simulink model "MSDR_and_BOP_v1_1"  (R2019a)
settings: Solver=ode45  StartTime=0.0  StopTime=15000  FixedStep=0.1  MaxStep=10
values from neighbouring files (symbols this model uses):
  a_f = -3.22E-5    (= -3.22e-05)    [MSDR_parameters_v1_1.m]
  a_g = +2.35E-5    (= 2.35e-05)    [MSDR_parameters_v1_1.m]
  A_s = 1.2245    [MSDR_parameters_v1_1.m]
  beta = [0.000223, 0.001457, 0.001307, 0.002628, 0.000766, 0.000280]    [MSDR_parameters_v1_1.m]
  beta_t = sum(beta)    [MSDR_parameters_v1_1.m]
  ce1 = 1.2471e-07    [MSDR_parameters_v1_1.m]
  ce2 = 5.3816e-14    [MSDR_parameters_v1_1.m]
  ce3 = 3.3721e-08    [MSDR_parameters_v1_1.m]
  Cp_fw = 3200.448e-6    (= 0.003200448)    [MSDR_parameters_v1_1.m]
  Cp_hr = 0.0021520    (= 0.002152)    [MSDR_parameters_v1_1.m]
  Cp_p = Cp_s_shx    (= 0.00154912)    [MSDR_parameters_v1_1.m]
  Cp_s = Cp_s*1e-6    (= 3.588208e-09)    [MSDR_parameters_v1_1.m]
  Cp_s_shx = 1549.12e-6    (= 0.00154912)    [MSDR_parameters_v1_1.m]
  Cp_sc = 4761.392e-6    (= 0.004761392)    [MSDR_parameters_v1_1.m]
  Cp_w = 456.056e-6    (= 0.000456056)    [MSDR_parameters_v1_1.m]
  D_it = 0.0141478    [MSDR_parameters_v1_1.m]
  D_ot = 0.015875    [MSDR_parameters_v1_1.m]
  dHs_dPs = -0.042433622114357    (= -0.0424336221144)    [MSDR_parameters_v1_1.m]
  eta_hp_isen = 0.861    [MSDR_parameters_v1_1.m]
  eta_lp_isen = 0.861    [MSDR_parameters_v1_1.m]
  gamma_I = 5.1135e-2    (= 0.051135)    [MSDR_parameters_v1_1.m]
  gamma_Xe = 1.1628e-2    (= 0.011628)    [MSDR_parameters_v1_1.m]
  H_fwh1 = 0.46009    [MSDR_parameters_v1_1.m]
  h_fwh1 = 0.5927    [MSDR_parameters_v1_1.m]
  H_fwh2 = 0.6784    [MSDR_parameters_v1_1.m]
  h_fwh2 = 0.5927    [MSDR_parameters_v1_1.m]
  H_lp_isen = 958.4*1054.35e-6/0.45359237    (= 2.22774699671)    [MSDR_parameters_v1_1.m]
  H_nc = 3.2952    [MSDR_parameters_v1_1.m]
  h_pw = h_s_shx    (= 0.00567446)    [MSDR_parameters_v1_1.m]
  H_rh = 2.8115    [MSDR_parameters_v1_1.m]
  h_wb = 13349.334646671E-6    (= 0.0133493346467)    [MSDR_parameters_v1_1.m]
  h_ws = 5732.378387768E-6    (= 0.00573237838777)    [MSDR_parameters_v1_1.m]
  h_wsc = 8385.005556375E-6    (= 0.00838500555638)    [MSDR_parameters_v1_1.m]
  hA_fg = [h_fg*A_fg/2, h_fg*A_fg/2]    [MSDR_parameters_v1_1.m]
  hA_p_phx1 = h_p_phx*A_p_phx    [MSDR_parameters_v1_1.m]
  hA_p_phx2 = h_p_phx*A_p_phx    [MSDR_parameters_v1_1.m]
  hA_p_phx3 = h_p_phx*A_p_phx    [MSDR_parameters_v1_1.m]
  hA_p_phx4 = h_p_phx*A_p_phx    [MSDR_parameters_v1_1.m]
  hA_p_phx5 = h_p_phx*A_p_phx    [MSDR_parameters_v1_1.m]
  hA_p_phx6 = h_p_phx*A_p_phx    [MSDR_parameters_v1_1.m]
  hA_p_shx1 = h_p_shx*A_p_shx    [MSDR_parameters_v1_1.m]
  hA_p_shx2 = h_p_shx*A_p_shx    [MSDR_parameters_v1_1.m]
  hA_p_shx3 = h_p_shx*A_p_shx    [MSDR_parameters_v1_1.m]
  hA_p_shx4 = h_p_shx*A_p_shx    [MSDR_parameters_v1_1.m]
  hA_p_shx5 = h_p_shx*A_p_shx    [MSDR_parameters_v1_1.m]
  hA_p_shx6 = h_p_shx*A_p_shx    [MSDR_parameters_v1_1.m]
  hA_s_phx1 = h_s_phx*A_s_phx    [MSDR_parameters_v1_1.m]
  hA_s_phx2 = h_s_phx*A_s_phx    [MSDR_parameters_v1_1.m]
  hA_s_phx3 = h_s_phx*A_s_phx    [MSDR_parameters_v1_1.m]
  hA_s_phx4 = h_s_phx*A_s_phx    [MSDR_parameters_v1_1.m]
  hA_s_phx5 = h_s_phx*A_s_phx    [MSDR_parameters_v1_1.m]
  hA_s_phx6 = h_s_phx*A_s_phx    [MSDR_parameters_v1_1.m]
  hA_s_shx1 = h_s_shx*A_s_shx    [MSDR_parameters_v1_1.m]
  hA_s_shx2 = h_s_shx*A_s_shx    [MSDR_parameters_v1_1.m]
  hA_s_shx3 = h_s_shx*A_s_shx    [MSDR_parameters_v1_1.m]
  hA_s_shx4 = h_s_shx*A_s_shx    [MSDR_parameters_v1_1.m]
  hA_s_shx5 = h_s_shx*A_s_shx    [MSDR_parameters_v1_1.m]
  hA_s_shx6 = h_s_shx*A_s_shx    [MSDR_parameters_v1_1.m]
  I_0 = gamma_I*Sig_f_msdr*phi_0/lam_I    (= 4.38204721773e+16)    [MSDR_parameters_v1_1.m]
  Ifa = [0.25, 0.25]    [MSDR_parameters_v1_1.m]
  Ifb = [0.25, 0.25]    [MSDR_parameters_v1_1.m]
  Ig = [0.5, 0.5]    [MSDR_parameters_v1_1.m]
  K_1 = 11.632248097704855    (= 11.6322480977)    [MSDR_parameters_v1_1.m]
  K_4 = b(1)    [MSDR_parameters_v1_1.m]
  K_5 = a(1)    [MSDR_parameters_v1_1.m]
  K_b = 12.834854076292217    (= 12.8348540763)    [MSDR_parameters_v1_1.m]
  K_b_hp = 0.1634    [MSDR_parameters_v1_1.m]
  K_b_lp = 0.2174    [MSDR_parameters_v1_1.m]
  K_sc = -17.615718797133468    (= -17.6157187971)    [MSDR_parameters_v1_1.m]
  ka = [0.235, 0.235]    [MSDR_parameters_v1_1.m]
  kb = [0.235, 0.235]    [MSDR_parameters_v1_1.m]
  kga = [0.015, 0.015]    [MSDR_parameters_v1_1.m]
  kgb = [0.015, 0.015]    [MSDR_parameters_v1_1.m]
  L = 8.5344    [MSDR_parameters_v1_1.m]
  L_b = 2.3645    [MSDR_parameters_v1_1.m]
  L_s = 4.723    [MSDR_parameters_v1_1.m]
  Lam = 2.400E-04    (= 0.00024)    [MSDR_parameters_v1_1.m]
  lam = [0.0124, 0.0305, 0.111, 0.301, 1.14, 3.01]    [MSDR_parameters_v1_1.m]
  lam_bubl = 2.0e-2    (= 0.02)    [MSDR_parameters_v1_1.m]
  lam_I = 2.875e-5    (= 2.875e-05)    [MSDR_parameters_v1_1.m]
  lam_Xe = 2.0916e-5    (= 2.0916e-05)    [MSDR_parameters_v1_1.m]
  m_3m = W_3*2    (= 8618.207327)    [MSDR_parameters_v1_1.m]
  m_fm = W_f*2    (= 9978.96)    [MSDR_parameters_v1_1.m]
  m_sb = 1717    [MSDR_parameters_v1_1.m]
  M_stm = 0.018    [MSDR_parameters_v1_1.m]
  mb_cpb = 2.689619410657651e+00    (= 2.68961941066)    [MSDR_parameters_v1_1.m]
  mcp_fa = mfa*Cp_f    [MSDR_parameters_v1_1.m]
  mcp_fb = mfb*Cp_f    [MSDR_parameters_v1_1.m]
  mcp_g = mg*Cp_g    [MSDR_parameters_v1_1.m]
  mcp_p_phx1 = Cp_p_phx*mp_phx1    [MSDR_parameters_v1_1.m]
  mcp_p_phx2 = Cp_p_phx*mp_phx2    [MSDR_parameters_v1_1.m]
  mcp_p_phx3 = Cp_p_phx*mp_phx3    [MSDR_parameters_v1_1.m]
  mcp_p_phx4 = Cp_p_phx*mp_phx4    [MSDR_parameters_v1_1.m]
  mcp_p_phx5 = Cp_p_phx*mp_phx5    [MSDR_parameters_v1_1.m]
  mcp_p_phx6 = Cp_p_phx*mp_phx6    [MSDR_parameters_v1_1.m]
  mcp_p_shx1 = Cp_p_shx*mp_shx1    [MSDR_parameters_v1_1.m]
  mcp_p_shx2 = Cp_p_shx*mp_shx2    [MSDR_parameters_v1_1.m]
  mcp_p_shx3 = Cp_p_shx*mp_shx3    [MSDR_parameters_v1_1.m]
  mcp_p_shx4 = Cp_p_shx*mp_shx4    [MSDR_parameters_v1_1.m]
  mcp_p_shx5 = Cp_p_shx*mp_shx5    [MSDR_parameters_v1_1.m]
  mcp_p_shx6 = Cp_p_shx*mp_shx6    [MSDR_parameters_v1_1.m]
  mcp_s_phx1 = Cp_s_phx*ms_phx1    [MSDR_parameters_v1_1.m]
  mcp_s_phx2 = Cp_s_phx*ms_phx2    [MSDR_parameters_v1_1.m]
  mcp_s_phx3 = Cp_s_phx*ms_phx3    [MSDR_parameters_v1_1.m]
  mcp_s_phx4 = Cp_s_phx*ms_phx4    [MSDR_parameters_v1_1.m]
  mcp_s_phx5 = Cp_s_phx*ms_phx5    [MSDR_parameters_v1_1.m]
  mcp_s_phx6 = Cp_s_phx*ms_phx6    [MSDR_parameters_v1_1.m]
  mcp_s_shx1 = Cp_s_shx*ms_shx1    [MSDR_parameters_v1_1.m]
  mcp_s_shx2 = Cp_s_shx*ms_shx1    [MSDR_parameters_v1_1.m]
  mcp_s_shx3 = Cp_s_shx*ms_shx1    [MSDR_parameters_v1_1.m]
  mcp_s_shx4 = Cp_s_shx*ms_shx1    [MSDR_parameters_v1_1.m]
  mcp_s_shx5 = Cp_s_shx*ms_shx1    [MSDR_parameters_v1_1.m]
  mcp_s_shx6 = Cp_s_shx*ms_shx1    [MSDR_parameters_v1_1.m]
  mcp_t_phx1 = Cp_t_phx*mt_phx1    [MSDR_parameters_v1_1.m]
  mcp_t_phx2 = Cp_t_phx*mt_phx2    [MSDR_parameters_v1_1.m]
  mcp_t_phx3 = Cp_t_phx*mt_phx3    [MSDR_parameters_v1_1.m]
  mcp_t_phx4 = Cp_t_phx*mt_phx4    [MSDR_parameters_v1_1.m]
  mcp_t_phx5 = Cp_t_phx*mt_phx5    [MSDR_parameters_v1_1.m]
  mcp_t_phx6 = Cp_t_phx*mt_phx6    [MSDR_parameters_v1_1.m]
  mcp_t_shx1 = Cp_t_phx*mt_shx1    [MSDR_parameters_v1_1.m]
  ... (+177 more)
undefined symbols (not defined in the file or in its folder): C0, H_con_table, H_convap_table, H_rh_table, H_rh_table1, H_rh_table2, H_rhvap_table, H_s_table, H_table, hA_p_thx1, hA_p_thx2, hA_p_thx3, hA_s_thx1, hA_s_thx2, hA_s_thx3, ln, mcp_p_thx1, mcp_p_thx2, mcp_p_thx3, mcp_s_thx1, mcp_s_thx2, mcp_s_thx3, mcp_t_thx1, mcp_t_thx2, mcp_t_thx3, mp_thx1, mp_thx2, mp_thx3, ms_thx1, ms_thx2, ms_thx3, P_con_table, P_nc_table, P_rh_table, P_rh_table1, pres_table, rho_rh_table, rho_table, SV_nc_table, T0_p_thx1, T0_p_thx2, T0_p_thx3, T0_s_thx1, T0_s_thx2, T0_s_thx3, T0_t_thx1, T0_t_thx2, T0_t_thx3, temp_table, u14, Wp_thx1, Wp_thx2, Wp_thx3, Ws_thx1, Ws_thx2, Ws_thx3
libraries: simulink x10
(part 4 of 4)

== system MSDR_and_BOP_v1_1/HEAT EXCHANGERS/HEAT EXCHANGER LOOP 6/THX2 HEAT TRANSFER ==
  PRIMARY FLUID INLET TEMPERATURE : Inport
  SECONDARY FLUID INLET TEMPERATURE : Inport  Port=2
  PRIMARY FLOW FRACTION : Inport  Port=3
  PRIMARY HEAT TRANSFER FRACTION : Inport  Port=4
  SECONDARY FLOW FRACTION : Inport  Port=5
  SECONDARY HEAT TRANSFER FRACTION : Inport  Port=6
  Mux : Mux  Inputs=16
      settings: DisplayOption=signals
  To Workspace : ToWorkspace  VariableName=thx3_ht  SampleTime=-1
  Tp1_thx3 : Integrator  InitialCondition=T0_p_thx3(1)
  Tp2_thx3 : Integrator  InitialCondition=T0_p_thx3(2)
  "Tp3_thx3 " : Integrator  InitialCondition=T0_p_thx3(3)
  Tp4_thx3 : Integrator  InitialCondition=T0_p_thx3(4)
  Ts1_thx3 : Integrator  InitialCondition=T0_s_thx3(1)
  Ts2_thx3 : Integrator  InitialCondition=T0_s_thx3(2)
  Ts3_thx3 : Integrator  InitialCondition=T0_s_thx3(3)
  Ts4_thx3 : Integrator  InitialCondition=T0_s_thx3(4)
  Tt1_thx3 : Integrator  InitialCondition=T0_t_thx3(1)
  Tt2_thx3 : Integrator  InitialCondition=T0_t_thx3(2)
  d(Tp1_thx3)/dt : Fcn  Expr=(u[13]*Wp_thx3/mp_thx3(1))*(u[1] - u[3]) + (u[14]*hA_p_thx3(1)/mcp_p_thx3(1))*(u[7] - u[3])
  d(Tp2_thx3)/dt : Fcn  Expr=(u[13]*Wp_thx3/mp_thx3(2))*(u[3] - u[4]) + (u[14]*hA_p_thx3(2)/mcp_p_thx3(2))*(u[7] - u[3])
  d(Tp3_thx3)/dt : Fcn  Expr=(u[13]*Wp_thx3/mp_thx3(3))*(u[4] - u[5]) + (u[14]*hA_p_thx3(3)/mcp_p_thx3(3))*(u[8] - u[5])
  d(Tp4_thx3)/dt : Fcn  Expr=(u[13]*Wp_thx3/mp_thx3(4))*(u[5] - u[6]) + (u[14]*hA_p_thx3(4)/mcp_p_thx3(4))*(u[8] - u[5])
  d(Ts1_thx3)/dt : Fcn  Expr=(u[15]*Ws_thx3/ms_thx3(1))*(u[2] - u[9]) + (u[16]*hA_s_thx3(1)/mcp_s_thx3(1))*(u[8] - u[9])
  d(Ts2_thx3)/dt : Fcn  Expr=(u[15]*Ws_thx3/ms_thx3(2))*(u[9] - u[10]) + (u[16]*hA_s_thx3(2)/mcp_s_thx3(2))*(u[8] - u[9])
  d(Ts3_thx3)/dt : Fcn  Expr=(u[15]*Ws_thx3/ms_thx3(3))*(u[10] - u[11]) + (u[16]*hA_s_thx3(3)/mcp_s_thx3(3))*(u[7] - u[11])
  d(Ts4_thx3)/dt : Fcn  Expr=(u[15]*Ws_thx3/ms_thx3(4))*(u[11] - u[12]) + (u[16]*hA_s_thx3(4)/mcp_s_thx3(4))*(u[7] - u[11])
  d(Tt1_thx3)/dt : Fcn  Expr=(u[14]*(hA_p_thx3(1) + hA_p_thx3(2))/mcp_t_thx3(1))*(u[3] - u[7]) + (u[16]*(hA_s_thx3(1) + hA_s_thx3(2))/mcp_t_thx3(1))*(u[11] - u[7])
  d(Tt2_thx3)/dt : Fcn  Expr=(u[14]*(hA_p_thx3(3) + hA_p_thx3(4))/mcp_t_thx3(2))*(u[5] - u[8]) + (u[16]*(hA_s_thx3(3) + hA_s_thx3(4))/mcp_t_thx3(2))*(u[9] - u[8])
  THX3 TEMPERATURES : Outport
  wires:
  Ts1_thx3/1 -> Mux/9
  Ts2_thx3/1 -> Mux/10
  d(Ts2_thx3)/dt/1 -> Ts2_thx3/1
  d(Tp4_thx3)/dt/1 -> Tp4_thx3/1
  Tt1_thx3/1 -> Mux/7
  d(Tp2_thx3)/dt/1 -> Tp2_thx3/1
  Tp4_thx3/1 -> Mux/6
  d(Tt2_thx3)/dt/1 -> Tt2_thx3/1
  SECONDARY FLUID INLET TEMPERATURE/1 -> Mux/2
  Tt2_thx3/1 -> Mux/8
  Mux/1 -> To Workspace/1, THX3 TEMPERATURES/1, d(Ts4_thx3)/dt/1, d(Ts3_thx3)/dt/1, d(Ts2_thx3)/dt/1, d(Ts1_thx3)/dt/1, d(Tt2_thx3)/dt/1, d(Tt1_thx3)/dt/1, d(Tp4_thx3)/dt/1, d(Tp3_thx3)/dt/1, d(Tp2_thx3)/dt/1, d(Tp1_thx3)/dt/1
  d(Tp1_thx3)/dt/1 -> Tp1_thx3/1
  d(Ts4_thx3)/dt/1 -> Ts4_thx3/1
  Tp1_thx3/1 -> Mux/3
  d(Ts1_thx3)/dt/1 -> Ts1_thx3/1
  d(Ts3_thx3)/dt/1 -> Ts3_thx3/1
  Ts3_thx3/1 -> Mux/11
  Ts4_thx3/1 -> Mux/12
  "Tp3_thx3 "/1 -> Mux/5
  d(Tp3_thx3)/dt/1 -> "Tp3_thx3 "/1
  Tp2_thx3/1 -> Mux/4
  d(Tt1_thx3)/dt/1 -> Tt1_thx3/1
  PRIMARY FLUID INLET TEMPERATURE/1 -> Mux/1
  SECONDARY HEAT TRANSFER FRACTION/1 -> Mux/16
  PRIMARY FLOW FRACTION/1 -> Mux/13
  PRIMARY HEAT TRANSFER FRACTION/1 -> Mux/14
  SECONDARY FLOW FRACTION/1 -> Mux/15

== system MSDR_and_BOP_v1_1/HEAT EXCHANGERS/HEAT EXCHANGER LOOP 6/THX3 MATERIAL TRANSPORT ==
  THX3 TEMPERATURES : Inport
  wires:
  THX3 TEMPERATURES/1 -> ?

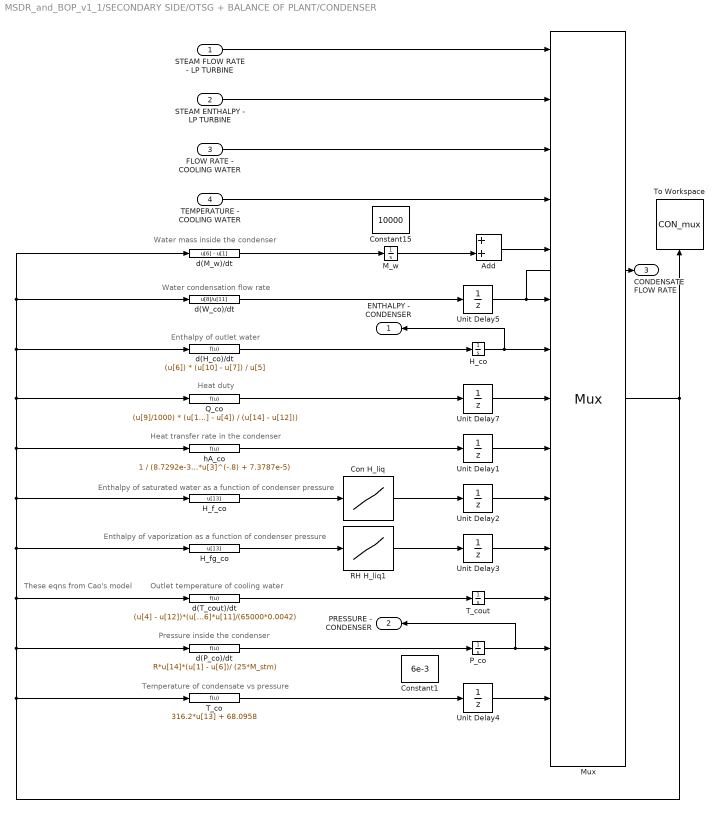
== system MSDR_and_BOP_v1_1/SECONDARY SIDE/OTSG + BALANCE OF PLANT/CONDENSER ==
  note: Water mass inside the condenser
  note: Water condensation flow rate
  note: Enthalpy of outlet water
  note: Heat duty
  note: Heat transfer rate in the condenser
  note: Enthalpy of saturated water as a function of condenser pressure
  note: Enthalpy of vaporization as a function of condenser pressure
  note: Outlet temperature of cooling water
  note: Pressure inside the condenser
  note: Temperature of condensate vs pressure
  note: These eqns from Cao's model
  STEAM FLOW RATE - LP TURBINE : Inport
  STEAM ENTHALPY - LP TURBINE : Inport  Port=2
  FLOW RATE - COOLING WATER : Inport  Port=3
  TEMPERATURE - COOLING WATER : Inport  Port=4
  Add : Sum
  Con H_liq : Lookup_n-D  NumberOfTableDimensions=1  BreakpointsForDimension1=P_con_table  Table=H_con_table  InternalRulePriority=Speed  RndMeth=Simplest  InputSameDT=on
  Constant1 : Constant  Value=6e-3
  Constant15 : Constant  Value=10000
  H_co : Integrator  InitialCondition=.149
  H_f_co : Fcn  Expr=u[13]
  H_fg_co : Fcn  Expr=u[13]
  M_w : Integrator  InitialCondition=10000
  Mux : Mux  Inputs=15
      settings: DisplayOption=signals
  P_co : Integrator  InitialCondition=0.006
  Q_co : Fcn  Expr=(u[9]/1000) * (u[12] - u[4]) / ln((u[14] - u[4]) / (u[14] - u[12]))
  RH H_liq1 : Lookup_n-D  NumberOfTableDimensions=1  BreakpointsForDimension1=P_con_table  Table=H_convap_table  InternalRulePriority=Speed  RndMeth=Simplest  InputSameDT=on
  T_co : Fcn  Expr=316.2*u[13] + 68.0958
  T_cout : Integrator  InitialCondition=40
  To Workspace : ToWorkspace  VariableName=CON_mux  SampleTime=0.1
      settings: Save2DSignal=2-D array (concatenate along first dimension)
  Unit Delay1 : UnitDelay  InitialCondition=140  SampleTime=-1  HasFrameUpgradeWarning=on
  Unit Delay2 : UnitDelay  InitialCondition=0.149  SampleTime=-1  HasFrameUpgradeWarning=on
  Unit Delay3 : UnitDelay  InitialCondition=2.35  SampleTime=-1  HasFrameUpgradeWarning=on
  Unit Delay4 : UnitDelay  InitialCondition=90  SampleTime=-1  HasFrameUpgradeWarning=on
  Unit Delay5 : UnitDelay  InitialCondition=159  SampleTime=-1  HasFrameUpgradeWarning=on
  Unit Delay7 : UnitDelay  InitialCondition=375  SampleTime=-1  HasFrameUpgradeWarning=on
  d(H_co)/dt : Fcn  Expr=(u[6]) * (u[10] - u[7]) / u[5]
  d(M_w)/dt : Fcn  Expr=u[6] - u[1]
  d(P_co)/dt : Fcn  Expr=R*u[14]*(u[1] - u[6])/ (25*M_stm)
  d(T_cout)/dt : Fcn  Expr=(u[4] - u[12])*(u[3]/65000) + u[6]*u[11]/(65000*0.0042)
  d(W_co)/dt : Fcn  Expr=u[8]/u[11]
  hA_co : Fcn  Expr=1 / (8.7292e-3*u[3]^(-.8) + 7.3787e-5)
  ENTHALPY - CONDENSER : Outport
  PRESSURE - CONDENSER : Outport  Port=2
  CONDENSATE FLOW RATE : Outport  Port=3
  wires:
  STEAM FLOW RATE - LP TURBINE/1 -> Mux/1
  d(M_w)/dt/1 -> M_w/1
  STEAM ENTHALPY - LP TURBINE/1 -> Mux/2
  FLOW RATE - COOLING WATER/1 -> Mux/3
  TEMPERATURE - COOLING WATER/1 -> Mux/4
  d(W_co)/dt/1 -> Unit Delay5/1
  Unit Delay5/1 -> CONDENSATE FLOW RATE/1, Mux/6
  d(H_co)/dt/1 -> H_co/1
  H_co/1 -> ENTHALPY - CONDENSER/1, Mux/7
  Unit Delay7/1 -> Mux/8
  Q_co/1 -> Unit Delay7/1
  Unit Delay1/1 -> Mux/9
  hA_co/1 -> Unit Delay1/1
  Unit Delay2/1 -> Mux/10
  H_fg_co/1 -> RH H_liq1/1
  Unit Delay3/1 -> Mux/11
  d(T_cout)/dt/1 -> T_cout/1
  T_cout/1 -> Mux/12
  P_co/1 -> Mux/13, PRESSURE - CONDENSER/1
  d(P_co)/dt/1 -> P_co/1
  Mux/1 -> To Workspace/1, T_co/1, d(P_co)/dt/1, H_fg_co/1, H_f_co/1, hA_co/1, Q_co/1, d(H_co)/dt/1, d(W_co)/dt/1, d(M_w)/dt/1, d(T_cout)/dt/1
  Unit Delay4/1 -> Mux/14
  T_co/1 -> Unit Delay4/1
  M_w/1 -> Add/2
  Add/1 -> Mux/5
  Con H_liq/1 -> Unit Delay2/1
  H_f_co/1 -> Con H_liq/1
  RH H_liq1/1 -> Unit Delay3/1

== system MSDR_and_BOP_v1_1/SECONDARY SIDE/OTSG + BALANCE OF PLANT/FEEDWATER HEATER 1 - LOW-PRESSURE ==
  note: Enthalpy of feedwater heater 1
  note: Heat transfer rate in the feedwater heater 1
  STEAM FLOW RATE - LP TURBINE : Inport
  STEAM BLEED FLOW - LP TURBINE : Inport  Port=2
  FLOW from FWH2 : Inport  Port=3
  ENTHALPY - CONDENSER : Inport  Port=4
  H'_fwh : Integrator  InitialCondition=H_fwh1
  Mux : Mux  Inputs=7
      settings: DisplayOption=signals
  Q_fwh1 : Fcn  Expr=h_fwh1*(u[3] + u[2])
  To Workspace : ToWorkspace  VariableName=FWH1_mux  SampleTime=0.1
      settings: Save2DSignal=2-D array (concatenate along first dimension)
  Unit Delay1 : UnitDelay  InitialCondition=W_fw  SampleTime=-1  HasFrameUpgradeWarning=on
  Unit Delay7 : UnitDelay  InitialCondition=96.368  SampleTime=-1  HasFrameUpgradeWarning=on
  W_fw : Fcn  Expr=u[1] + u[2] + u[3]
  d(H'_fwh)/dt : Fcn  Expr=u[6]/(tau_fwh1*u[7]) + (u[4] - u[5])/tau_fwh1
  ENTHALPY - FWH1 : Outport
  FEEDWATER FLOW RATE : Outport  Port=2
  wires:
  STEAM FLOW RATE - LP TURBINE/1 -> Mux/1
  STEAM BLEED FLOW - LP TURBINE/1 -> Mux/2
  FLOW from FWH2/1 -> Mux/3
  Mux/1 -> To Workspace/1, W_fw/1, Q_fwh1/1, d(H'_fwh)/dt/1
  ENTHALPY - CONDENSER/1 -> Mux/4
  d(H'_fwh)/dt/1 -> H'_fwh/1
  H'_fwh/1 -> Mux/5, ENTHALPY - FWH1/1
  Q_fwh1/1 -> Unit Delay7/1
  Unit Delay7/1 -> Mux/6
  W_fw/1 -> Unit Delay1/1
  Unit Delay1/1 -> FEEDWATER FLOW RATE/1, Mux/7

== system MSDR_and_BOP_v1_1/SECONDARY SIDE/OTSG + BALANCE OF PLANT/FEEDWATER HEATER 2 - HIGH-PRESSURE ==
  note: Enthalpy of feedwater heater 2
  note: Heat transfer rate in the feedwater heater 2
  note: Flow to FWH1
  note: Temperature of feedwater after heating
  STEAM BLEED FLOW - HP TURBINE : Inport
  FLOW from MOISTURE SEPARATOR : Inport  Port=2
  FLOW from REHEATER : Inport  Port=3
  FLOW from MS to RH : Inport  Port=4
  FLOW from FWH1 : Inport  Port=5
  ENTHALPY - FWH1 : Inport  Port=6
  STEAM FLOW RATE - NOZZLE CHEST : Inport  Port=7
  H_fwh : Integrator  InitialCondition=H_fwh2
  Mux : Mux  Inputs=11
      settings: DisplayOption=signals
  Q_fwh2 : Fcn  Expr=h_fwh2*(u[1] + u[2] + u[3])
  T_fw : Integrator  InitialCondition=205.58
  To Workspace : ToWorkspace  VariableName=FWH2_mux  SampleTime=0.1
      settings: Save2DSignal=2-D array (concatenate along first dimension)
  Unit Delay7 : UnitDelay  InitialCondition=70.197  SampleTime=-1  HasFrameUpgradeWarning=on
  d(H_fwh)/dt : Fcn  Expr=u[9]/(tau_fwh2*u[5]) + (u[6] - u[8])/tau_fwh2
  d(T_fw)/dt : Fcn  Expr=(u[9]/(tau_fwh2*u[5]) + (u[6] - Cp_fw*u[11])/tau_fwh2) / Cp_fw
  d(w'_fwh)/dt : Fcn  Expr=(u[1] + u[2] + u[3] - u[10])/tau_rh2
  w'_fwh : Integrator  InitialCondition=118.44
  ENTHALPY - FWH2 : Outport
  FLOW to FWH1 : Outport  Port=2
  FEEDWATER FLOW RATE : Outport  Port=3
  TEMPERATURE - FEEDWATER : Outport  Port=4
  wires:
  STEAM BLEED FLOW - HP TURBINE/1 -> Mux/1
  FLOW from MOISTURE SEPARATOR/1 -> Mux/2
  FLOW from REHEATER/1 -> Mux/3
  FLOW from MS to RH/1 -> Mux/4
  d(H_fwh)/dt/1 -> H_fwh/1
  H_fwh/1 -> Mux/8, ENTHALPY - FWH2/1
  Q_fwh2/1 -> Unit Delay7/1
  Unit Delay7/1 -> Mux/9
  FLOW from FWH1/1 -> FEEDWATER FLOW RATE/1, Mux/5
  ENTHALPY - FWH1/1 -> Mux/6
  STEAM FLOW RATE - NOZZLE CHEST/1 -> Mux/7
  d(w'_fwh)/dt/1 -> w'_fwh/1
  w'_fwh/1 -> Mux/10, FLOW to FWH1/1
  d(T_fw)/dt/1 -> T_fw/1
  T_fw/1 -> Mux/11, TEMPERATURE - FEEDWATER/1
  Mux/1 -> To Workspace/1, d(T_fw)/dt/1, d(w'_fwh)/dt/1, Q_fwh2/1, d(H_fwh)/dt/1

== system MSDR_and_BOP_v1_1/SECONDARY SIDE/OTSG + BALANCE OF PLANT/HIGH PRESSURE TURBINE ==
  note: Steam flow from HP turbine to moisture separator
  note: HP turbine bleed flow rate to feed water heater 2
  note: Enthalpy of steam at moisture separator
  note: Enthalpy of steam at isentropic endpoints from pressure P_nc
  STEAM FLOW RATE - NOZZLE CHEST : Inport
  STEAM ENTHALPY - NOZZLE CHEST : Inport  Port=2
  STEAM PRESSURE - NOZZLE CHEST : Inport  Port=3
  STEAM PRESSURE - REHEATER : Inport  Port=4
  H_hp : Fcn  Expr=(u[8] - u[2])*eta_hp_isen + u[2]
  H_hp_isen : Fcn  Expr=term1 + ce1*(u[4] - p1) - ce2*(u[4] - p1)^2 - ce3*(u[3] - p2)
  Mux : Mux  Inputs=8
      settings: DisplayOption=signals
  To Workspace : ToWorkspace  VariableName=HPT_mux  SampleTime=0.1
      settings: Save2DSignal=2-D array (concatenate along first dimension)
  Unit Delay1 : UnitDelay  InitialCondition=2.6201  SampleTime=-1  HasFrameUpgradeWarning=on
  Unit Delay2 : UnitDelay  InitialCondition=2.5111  SampleTime=-1  HasFrameUpgradeWarning=on
  Unit Delay3 : UnitDelay  InitialCondition=44.134  SampleTime=-1  HasFrameUpgradeWarning=on
  d(w''_2)/dt : Fcn  Expr=((u[1] - u[6]) - u[5])/tau_hp
  w''_2 : Integrator  InitialCondition=w_hp_out
  w_b_hp : Fcn  Expr=K_b_hp*u[1]
  STEAM FLOW RATE - HP TURBINE : Outport
  STEAM BLEED FLOW - HP TURBINE : Outport  Port=2
  STEAM ENTHALPY - HP TURBINE : Outport  Port=3
  wires:
  STEAM FLOW RATE - NOZZLE CHEST/1 -> Mux/1
  STEAM ENTHALPY - NOZZLE CHEST/1 -> Mux/2
  STEAM PRESSURE - NOZZLE CHEST/1 -> Mux/3
  STEAM PRESSURE - REHEATER/1 -> Mux/4
  d(w''_2)/dt/1 -> w''_2/1
  w_b_hp/1 -> Unit Delay3/1
  H_hp/1 -> Unit Delay1/1
  H_hp_isen/1 -> Unit Delay2/1
  w''_2/1 -> STEAM FLOW RATE - HP TURBINE/1, Mux/5
  Mux/1 -> To Workspace/1, H_hp_isen/1, H_hp/1, w_b_hp/1, d(w''_2)/dt/1
  Unit Delay3/1 -> STEAM BLEED FLOW - HP TURBINE/1, Mux/6
  Unit Delay1/1 -> STEAM ENTHALPY - HP TURBINE/1, Mux/7
  Unit Delay2/1 -> Mux/8

== system MSDR_and_BOP_v1_1/SECONDARY SIDE/OTSG + BALANCE OF PLANT/LOW PRESSURE TURBINE ==
  note: Steam flow from HP turbine to moisture separator
  FLOW from REHEATER : Inport
  STEAM ENTHALPY - REHEATER : Inport  Port=2
  H_lp : Fcn  Expr=u[2] - eta_lp_isen*(u[2] - H_lp_isen)
  Mux : Mux  Inputs=5
      settings: DisplayOption=signals
  To Workspace : ToWorkspace  VariableName=LPT_mux  SampleTime=0.1
      settings: Save2DSignal=2-D array (concatenate along first dimension)
  Unit Delay1 : UnitDelay  InitialCondition=2.3089  SampleTime=-1  HasFrameUpgradeWarning=on
  Unit Delay3 : UnitDelay  InitialCondition=44.156  SampleTime=-1  HasFrameUpgradeWarning=on
  d(w'_3)/dt : Fcn  Expr=((u[1] - u[4]) - u[3])/tau_lp
  w'_3 : Integrator  InitialCondition=w_lp_out
  w_b_lp : Fcn  Expr=K_b_lp*u[1]
  STEAM FLOW RATE - LP TURBINE : Outport
  STEAM BLEED FLOW - LP TURBINE : Outport  Port=2
  STEAM ENTHALPY - LP TURBINE : Outport  Port=3
  wires:
  FLOW from REHEATER/1 -> Mux/1
  STEAM ENTHALPY - REHEATER/1 -> Mux/2
  w'_3/1 -> STEAM FLOW RATE - LP TURBINE/1, Mux/3
  d(w'_3)/dt/1 -> w'_3/1
  w_b_lp/1 -> Unit Delay3/1
  Mux/1 -> To Workspace/1, H_lp/1, w_b_lp/1, d(w'_3)/dt/1
  Unit Delay3/1 -> STEAM BLEED FLOW - LP TURBINE/1, Mux/4
  Unit Delay1/1 -> Mux/5, STEAM ENTHALPY - LP TURBINE/1
  H_lp/1 -> Unit Delay1/1

== system MSDR_and_BOP_v1_1/SECONDARY SIDE/OTSG + BALANCE OF PLANT/MOISTURE SEPARATOR ==
  note: Steam flow from moisture separator to reheater
  note: Steam flow from moisture separator to feedwater heater2
  ENTHALPY OF VAPORIZATION : Inport
  ENTHALPY OF REHEATER FEEDWATER : Inport  Port=2
  STEAM FLOW RATE - NOZZLE CHEST : Inport  Port=3
  STEAM FLOW RATE - HP TURBINE : Inport  Port=4
  STEAM BLEED FLOW - HP TURBINE : Inport  Port=5
  STEAM ENTHALPY - HP TURBINE : Inport  Port=6
  Mux : Mux  Inputs=8
      settings: DisplayOption=signals
  To Workspace : ToWorkspace  VariableName=MS_mux  SampleTime=0.1
      settings: Save2DSignal=2-D array (concatenate along first dimension)
  w'_2 : Fcn  Expr=(u[6] - u[2])/u[1] * u[4]
  w_ms : Fcn  Expr=(u[3] - u[5]) - u[8]
  FLOW to HEATER2 : Outport
  FLOW to REHEATER : Outport  Port=2
  wires:
  ENTHALPY OF VAPORIZATION/1 -> Mux/1
  ENTHALPY OF REHEATER FEEDWATER/1 -> Mux/2
  STEAM FLOW RATE - NOZZLE CHEST/1 -> Mux/3
  STEAM FLOW RATE - HP TURBINE/1 -> Mux/4
  STEAM BLEED FLOW - HP TURBINE/1 -> Mux/5
  STEAM ENTHALPY - HP TURBINE/1 -> Mux/6
  Mux/1 -> w'_2/1, w_ms/1, To Workspace/1
  w_ms/1 -> FLOW to HEATER2/1, Mux/7
  w'_2/1 -> FLOW to REHEATER/1, Mux/8

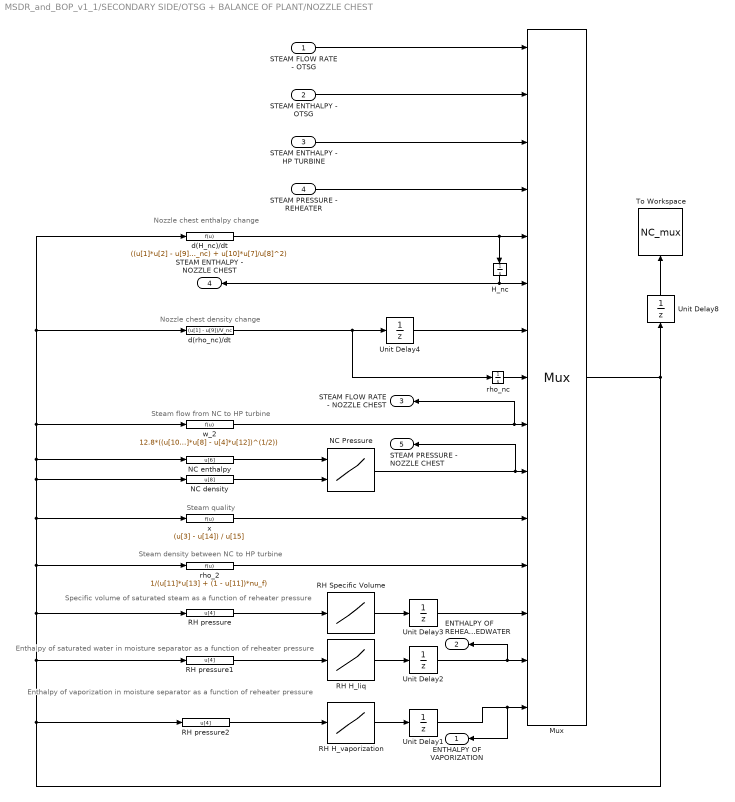
== system MSDR_and_BOP_v1_1/SECONDARY SIDE/OTSG + BALANCE OF PLANT/NOZZLE CHEST ==
  note: Nozzle chest density change
  note: Nozzle chest enthalpy change
  note: Steam flow from NC to HP turbine
  note: Steam quality
  note: Steam density between NC to HP turbine
  note: Specific volume of saturated steam as a function of reheater pressure
  note: Enthalpy of saturated water in moisture separator as a function of reheater pressure
  note: Enthalpy of vaporization in moisture separator as a function of reheater pressure
  STEAM FLOW RATE - OTSG : Inport
  STEAM ENTHALPY - OTSG : Inport  Port=2
  STEAM ENTHALPY - HP TURBINE : Inport  Port=3
  STEAM PRESSURE - REHEATER : Inport  Port=4
  H_nc : Integrator  InitialCondition=H_nc
  Mux : Mux  Inputs=15
      settings: DisplayOption=signals
  NC Pressure : Lookup_n-D  BreakpointsForDimension1=H_table  BreakpointsForDimension2=rho_table  Table=P_nc_table  InternalRulePriority=Speed  RndMeth=Simplest  InputSameDT=on
  NC density : Fcn  Expr=u[8]
  NC enthalpy : Fcn  Expr=u[6]
  RH H_liq : Lookup_n-D  NumberOfTableDimensions=1  BreakpointsForDimension1=P_rh_table1  Table=H_rh_table  InternalRulePriority=Speed  RndMeth=Simplest  InputSameDT=on
  RH H_vaporization : Lookup_n-D  NumberOfTableDimensions=1  BreakpointsForDimension1=P_rh_table1  Table=H_rhvap_table  InternalRulePriority=Speed  RndMeth=Simplest  InputSameDT=on
  RH Specific Volume : Lookup_n-D  NumberOfTableDimensions=1  BreakpointsForDimension1=P_rh_table1  Table=SV_nc_table  InternalRulePriority=Speed  RndMeth=Simplest  InputSameDT=on
  RH pressure : Fcn  Expr=u[4]
  RH pressure1 : Fcn  Expr=u[4]
  RH pressure2 : Fcn  Expr=u[4]
  To Workspace : ToWorkspace  VariableName=NC_mux  SampleTime=-1
      settings: Save2DSignal=2-D array (concatenate along first dimension)
  Unit Delay1 : UnitDelay  InitialCondition=1.8077  SampleTime=-1  HasFrameUpgradeWarning=on
  Unit Delay2 : UnitDelay  InitialCondition=.99522  SampleTime=-1  HasFrameUpgradeWarning=on
  Unit Delay3 : UnitDelay  InitialCondition=0.070431  SampleTime=-1  HasFrameUpgradeWarning=on
  Unit Delay4 : UnitDelay  SampleTime=-1  HasFrameUpgradeWarning=on
  Unit Delay8 : UnitDelay  InitialCondition=266.6348  SampleTime=-1  HasFrameUpgradeWarning=on
  d(H_nc)/dt : Fcn  Expr=((u[1]*u[2] - u[9]*u[6])/(u[8]*V_nc) + u[10]*u[7]/u[8]^2)
  d(rho_nc)/dt : Fcn  Expr=(u[1] - u[9])/V_nc
  rho_2 : Fcn  Expr=1/(u[11]*u[13] + (1 - u[11])*nu_f)
  rho_nc : Integrator  InitialCondition=74.07  UpperSaturationLimit=rho_nc
  w_2 : Fcn  Expr=12.8*((u[10]*u[8] - u[4]*u[12])^(1/2))
  x : Fcn  Expr=(u[3] - u[14]) / u[15]
  ENTHALPY OF VAPORIZATION : Outport
  ENTHALPY OF REHEATER FEEDWATER : Outport  Port=2
  STEAM FLOW RATE - NOZZLE CHEST : Outport  Port=3
  STEAM ENTHALPY - NOZZLE CHEST : Outport  Port=4
  STEAM PRESSURE - NOZZLE CHEST : Outport  Port=5
  wires:
  STEAM FLOW RATE - OTSG/1 -> Mux/1
  STEAM ENTHALPY - OTSG/1 -> Mux/2
  STEAM ENTHALPY - HP TURBINE/1 -> Mux/3
  STEAM PRESSURE - REHEATER/1 -> Mux/4
  H_nc/1 -> Mux/6, STEAM ENTHALPY - NOZZLE CHEST/1
  NC density/1 -> NC Pressure/2
  NC enthalpy/1 -> NC Pressure/1
  x/1 -> Mux/11
  Mux/1 -> RH pressure2/1, RH pressure1/1, RH pressure/1, rho_2/1, x/1, NC density/1, NC enthalpy/1, w_2/1, d(rho_nc)/dt/1, d(H_nc)/dt/1, Unit Delay8/1
  d(H_nc)/dt/1 -> Mux/5, H_nc/1
  w_2/1 -> STEAM FLOW RATE - NOZZLE CHEST/1, Mux/9
  NC Pressure/1 -> STEAM PRESSURE - NOZZLE CHEST/1, Mux/10
  Unit Delay8/1 -> To Workspace/1
  RH pressure2/1 -> RH H_vaporization/1
  RH pressure1/1 -> RH H_liq/1
  RH Specific Volume/1 -> Unit Delay3/1
  RH pressure/1 -> RH Specific Volume/1
  RH H_liq/1 -> Unit Delay2/1
  RH H_vaporization/1 -> Unit Delay1/1
  Unit Delay1/1 -> ENTHALPY OF VAPORIZATION/1, Mux/15
  rho_nc/1 -> Mux/8
  Unit Delay2/1 -> ENTHALPY OF REHEATER FEEDWATER/1, Mux/14
  Unit Delay3/1 -> Mux/13
  rho_2/1 -> Mux/12
  d(rho_nc)/dt/1 -> Unit Delay4/1, rho_nc/1
  Unit Delay4/1 -> Mux/7

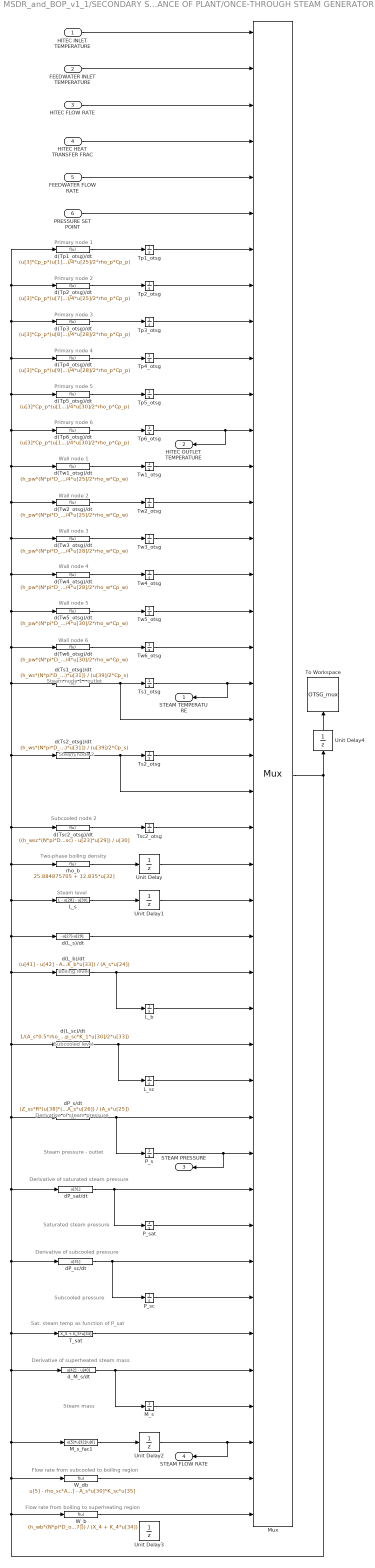
== system MSDR_and_BOP_v1_1/SECONDARY SIDE/OTSG + BALANCE OF PLANT/ONCE-THROUGH STEAM GENERATOR ==
  note: Primary node 1
  note: Primary node 2
  note: Primary node 3
  note: Primary node 4
  note: Primary node 5
  note: Primary node 6
  note: Wall node 1
  note: Wall node 2
  note: Wall node 3
  note: Wall node 4
  note: Wall node 5
  note: Wall node 6
  note: Steam node 1 - outlet
  note: Steam level
  note: Boiling level
  note: Subcooled level
  note: Derivative of saturated steam pressure
  note: Sat. steam temp as function of P_sat
  note: Saturated steam pressure
  note: Subcooled pressure
  note: Derivative of steam pressure
  note: Derivative of subcooled pressure
  note: Steam pressure - outlet
  note: Subcooled node 2
  note: Steam node 2
  note: Two-phase boiling density
  note: Derivative of superheated steam mass
  note: Steam mass
  note: Flow rate from subcooled to boiling region
  note: Flow rate from boiling to superheating region
  HITEC INLET TEMPERATURE : Inport
  FEEDWATER INLET TEMPERATURE : Inport  Port=2
  HITEC FLOW RATE : Inport  Port=3
  HITEC HEAT TRANSFER FRAC : Inport  Port=4
  FEEDWATER FLOW RATE : Inport  Port=5
  PRESSURE SET POINT : Inport  Port=6
  L_b : Integrator  InitialCondition=L_b
  L_s : Fcn  Expr=L - u[28] - u[30]
  L_sc : Integrator  InitialCondition=.5344
  M_s : Integrator  InitialCondition=A_s*rho_s*L_s
  M_s_fac1 : Fcn  Expr=u[5]*u[32]/u[6]
  Mux : Mux  Inputs=42
      settings: DisplayOption=signals
  P_s : Integrator  InitialCondition=P_s
  P_sat : Integrator  InitialCondition=P_sat
  P_sc : Integrator  InitialCondition=P_sc
  T_sat : Fcn  Expr=X_5 + K_5*u[34]
  To Workspace : ToWorkspace  VariableName=OTSG_mux  SaveFormat=Timeseries  SampleTime=-1
  Tp1_otsg : Integrator  InitialCondition=T_p1
  Tp2_otsg : Integrator  InitialCondition=T_p2
  Tp3_otsg : Integrator  InitialCondition=T_p3
  Tp4_otsg : Integrator  InitialCondition=T_p4
  Tp5_otsg : Integrator  InitialCondition=T_p5
  Tp6_otsg : Integrator  InitialCondition=T_p6
  Ts1_otsg : Integrator  InitialCondition=T_s1
  Ts2_otsg : Integrator  InitialCondition=T_s2
  Tsc2_otsg : Integrator  InitialCondition=T_sc2
  Tw1_otsg : Integrator  InitialCondition=T_w1
  Tw2_otsg : Integrator  InitialCondition=T_w2
  Tw3_otsg : Integrator  InitialCondition=T_w3
  Tw4_otsg : Integrator  InitialCondition=T_w4
  Tw5_otsg : Integrator  InitialCondition=T_w5
  Tw6_otsg : Integrator  InitialCondition=T_w6
  Unit Delay : UnitDelay  InitialCondition=rho_b  SampleTime=-1  HasFrameUpgradeWarning=on
  Unit Delay1 : UnitDelay  InitialCondition=L_s  SampleTime=-1  HasFrameUpgradeWarning=on
  Unit Delay2 : UnitDelay  InitialCondition=W_fw  SampleTime=-1  HasFrameUpgradeWarning=on
  Unit Delay3 : UnitDelay  InitialCondition=W_fw  SampleTime=-1  HasFrameUpgradeWarning=on
  Unit Delay4 : UnitDelay  SampleTime=-1  HasFrameUpgradeWarning=on
  W_b : Fcn  Expr=(h_wb*(N*pi*D_ot*u[28])*(0.5*u[15] + 0.5*u[16] - u[37])) / (X_4 + K_4*u[34])
  W_db : Fcn  Expr=u[5] - rho_sc*A_s*u[29] - A_s*u[30]*K_sc*u[35]
  d(L_b)/dt : Fcn  Expr=(u[41] - u[42] - A_s*u[28]*K_b*u[33]) / (A_s*u[24])
  d(L_s)/dt : Fcn  Expr=-u[27]-u[29]
  d(L_sc)/dt : Fcn  Expr=1/(A_s*0.5*rho_sc*Cp_sc*(u[23] - u[37])) * (h_wsc*N*pi*D_ot*u[30]/2*(u[17] - u[37]) + Cp_sc*(u[5]*u[23] - (u[5] + u[41])*0.5*u[37]) - A_s*u[30]/2*(K_sc*Cp_sc*(u[23] - 2*u[37]) - 1)*u[35] - A_s*rho_sc*Cp_sc*K_1*u[30]/2*u[33])
  d(Tp1_otsg)/dt : Fcn  Expr=(u[3]*Cp_p*(u[1] - u[7]) + h_pw*(N*pi*D_it*u[25]/2)*(u[13] - u[7])) / (N*pi*(D_it^2)/4*u[25]/2*rho_p*Cp_p)
  d(Tp2_otsg)/dt : Fcn  Expr=(u[3]*Cp_p*(u[7] - u[8]) + h_pw*(N*pi*D_it*u[25]/2)*(u[14] - u[8])) / (N*pi*(D_it^2)/4*u[25]/2*rho_p*Cp_p)
  d(Tp3_otsg)/dt : Fcn  Expr=(u[3]*Cp_p*(u[8] - u[9]) + h_pw*(N*pi*D_it*u[28]/2)*(u[15] - u[9])) / (N*pi*(D_it^2)/4*u[28]/2*rho_p*Cp_p)
  d(Tp4_otsg)/dt : Fcn  Expr=(u[3]*Cp_p*(u[9] - u[10]) + h_pw*(N*pi*D_it*u[28]/2)*(u[16] - u[10])) / (N*pi*(D_it^2)/4*u[28]/2*rho_p*Cp_p)
  d(Tp5_otsg)/dt : Fcn  Expr=(u[3]*Cp_p*(u[10] - u[11]) + h_pw*(N*pi*D_it*u[30]/2)*(u[17] - u[11])) / (N*pi*(D_it^2)/4*u[30]/2*rho_p*Cp_p)
  d(Tp6_otsg)/dt : Fcn  Expr=(u[3]*Cp_p*(u[11] - u[12]) + h_pw*(N*pi*D_it*u[30]/2)*(u[18] - u[12])) / (N*pi*(D_it^2)/4*u[30]/2*rho_p*Cp_p)
  d(Ts1_otsg)/dt : Fcn  Expr=(h_ws*(N*pi*D_ot*u[25]/2)*(u[13] - u[19]) + u[40]*Cp_s*(u[21] - u[19]) + Cp_s*(u[21] - u[19])*u[38]/2 + (A_s*u[25]/2 - u[39]/2*dHs_dPs)*u[31]) / (u[39]/2*Cp_s)
  d(Ts2_otsg)/dt : Fcn  Expr=(h_ws*(N*pi*D_ot*u[25]/2)*(u[14] - u[21]) + u[42]*Cp_s*(u[37] - u[21]) + (A_s*u[25]/2 - u[39]/2*dHs_dPs)*u[31]) / (u[39]/2*Cp_s)
  d(Tsc2_otsg)/dt : Fcn  Expr=((h_wsc*(N*pi*D_ot*u[30]/2)*(u[18] - u[23]) + Cp_sc*(u[5]*u[2] - (u[5] + u[41])*0.5*u[23]) + A_s*u[30]/2*u[35]) * 2/(A_s*rho_sc*Cp_sc) - u[23]*u[29]) / u[30]
  d(Tw1_otsg)/dt : Fcn  Expr=(h_pw*(N*pi*D_it*u[25]/2)*(u[7] - u[13]) + h_ws*(N*pi*D_ot*u[25]/2)*(u[19] - u[13])) / (N*pi*(D_ot^2 - D_it^2)/4*u[25]/2*rho_w*Cp_w)
  d(Tw2_otsg)/dt : Fcn  Expr=(h_pw*(N*pi*D_it*u[25]/2)*(u[8] - u[14]) + h_ws*(N*pi*D_ot*u[25]/2)*(u[21] - u[14])) / (N*pi*(D_ot^2 - D_it^2)/4*u[25]/2*rho_w*Cp_w)
  d(Tw3_otsg)/dt : Fcn  Expr=(h_pw*(N*pi*D_it*u[28]/2)*(u[9] - u[15]) + h_wb*(N*pi*D_ot*u[28]/2)*(u[37] - u[15])) / (N*pi*(D_ot^2 - D_it^2)/4*u[28]/2*rho_w*Cp_w)
  d(Tw4_otsg)/dt : Fcn  Expr=(h_pw*(N*pi*D_it*u[28]/2)*(u[10] - u[16]) + h_wb*(N*pi*D_ot*u[28]/2)*(u[37] - u[16])) / (N*pi*(D_ot^2 - D_it^2)/4*u[28]/2*rho_w*Cp_w)
  d(Tw5_otsg)/dt : Fcn  Expr=(h_pw*(N*pi*D_it*u[30]/2)*(u[11] - u[17]) + h_wsc*(N*pi*D_ot*u[30]/2)*(u[37] - u[17])) / (N*pi*(D_ot^2 - D_it^2)/4*u[30]/2*rho_w*Cp_w)
  d(Tw6_otsg)/dt : Fcn  Expr=(h_pw*(N*pi*D_it*u[30]/2)*(u[12] - u[18]) + h_wsc*(N*pi*D_ot*u[30]/2)*(u[23] - u[18])) / (N*pi*(D_ot^2 - D_it^2)/4*u[30]/2*rho_w*Cp_w)
  dP_s/dt : Fcn  Expr=(Z_ss*R*(u[38]*(u[19] + u[21]) + u[39]*(u[20] + u[22]))/(2*M_stm) - u[32]*A_s*u[26]) / (A_s*u[25])
  dP_sat/dt : Fcn  Expr=u[31]
  dP_sc/dt : Fcn  Expr=u[31]
  d_M_s/dt : Fcn  Expr=u[42] - u[40]
  rho_b : Fcn  Expr=25.884875705 + 12.835*u[32]
  STEAM TEMPERATURE : Outport
  HITEC OUTLET TEMPERATURE : Outport  Port=2
  STEAM PRESSURE : Outport  Port=3
  STEAM FLOW RATE : Outport  Port=4
  wires:
  FEEDWATER INLET TEMPERATURE/1 -> Mux/2
  d(Tp1_otsg)/dt/1 -> Tp1_otsg/1
  HITEC INLET TEMPERATURE/1 -> Mux/1
  HITEC FLOW RATE/1 -> Mux/3
  HITEC HEAT TRANSFER FRAC/1 -> Mux/4
  FEEDWATER FLOW RATE/1 -> Mux/5
  PRESSURE SET POINT/1 -> Mux/6
  Tp1_otsg/1 -> Mux/7
  Tp2_otsg/1 -> Mux/8
  d(Tp2_otsg)/dt/1 -> Tp2_otsg/1
  Tp3_otsg/1 -> Mux/9
  d(Tp3_otsg)/dt/1 -> Tp3_otsg/1
  Tp4_otsg/1 -> Mux/10
  d(Tp4_otsg)/dt/1 -> Tp4_otsg/1
  Tp5_otsg/1 -> Mux/11
  d(Tp5_otsg)/dt/1 -> Tp5_otsg/1
  d(Tp6_otsg)/dt/1 -> Tp6_otsg/1
  Tp6_otsg/1 -> HITEC OUTLET TEMPERATURE/1, Mux/12
  Tw1_otsg/1 -> Mux/13
  d(Tw1_otsg)/dt/1 -> Tw1_otsg/1
  d(Tw2_otsg)/dt/1 -> Tw2_otsg/1
  Tw2_otsg/1 -> Mux/14
  Tw3_otsg/1 -> Mux/15
  d(Tw3_otsg)/dt/1 -> Tw3_otsg/1
  d(Tw4_otsg)/dt/1 -> Tw4_otsg/1
  Tw4_otsg/1 -> Mux/16
  Tw5_otsg/1 -> Mux/17
  d(Tw5_otsg)/dt/1 -> Tw5_otsg/1
  d(Tw6_otsg)/dt/1 -> Tw6_otsg/1
  Tw6_otsg/1 -> Mux/18
  Ts1_otsg/1 -> STEAM TEMPERATURE/1, Mux/19
  L_sc/1 -> Mux/30
  L_s/1 -> Unit Delay1/1
  L_b/1 -> Mux/28
  P_s/1 -> Mux/32, STEAM PRESSURE/1
  P_sat/1 -> Mux/34
  P_sc/1 -> Mux/36
  Tsc2_otsg/1 -> Mux/23
  d(Tsc2_otsg)/dt/1 -> Tsc2_otsg/1
  Ts2_otsg/1 -> Mux/21
  rho_b/1 -> Unit Delay/1
  Unit Delay/1 -> Mux/24
  M_s/1 -> Mux/39
  Mux/1 -> W_b/1, W_db/1, d_M_s/dt/1, T_sat/1, dP_sc/dt/1, dP_sat/dt/1, dP_s/dt/1, d(L_sc)/dt/1, d(L_b)/dt/1, d(L_s)/dt/1, L_s/1, rho_b/1, d(Tsc2_otsg)/dt/1, d(Ts2_otsg)/dt/1, d(Ts1_otsg)/dt/1, d(Tw6_otsg)/dt/1, d(Tw5_otsg)/dt/1, d(Tw4_otsg)/dt/1, d(Tw3_otsg)/dt/1, d(Tw2_otsg)/dt/1, d(Tw1_otsg)/dt/1, d(Tp6_otsg)/dt/1, d(Tp5_otsg)/dt/1, d(Tp4_otsg)/dt/1, d(Tp3_otsg)/dt/1, d(Tp2_otsg)/dt/1, d(Tp1_otsg)/dt/1, M_s_fac1/1, Unit Delay4/1
  d(Ts1_otsg)/dt/1 -> Mux/20, Ts1_otsg/1
  d(Ts2_otsg)/dt/1 -> Mux/22, Ts2_otsg/1
  dP_s/dt/1 -> Mux/31, P_s/1
  d(L_b)/dt/1 -> Mux/27, L_b/1
  d(L_s)/dt/1 -> Mux/26
  d(L_sc)/dt/1 -> Mux/29, L_sc/1
  dP_sat/dt/1 -> Mux/33, P_sat/1
  dP_sc/dt/1 -> Mux/35, P_sc/1
  Unit Delay1/1 -> Mux/25
  T_sat/1 -> Mux/37
  M_s_fac1/1 -> Unit Delay2/1
  d_M_s/dt/1 -> Mux/38, M_s/1
  Unit Delay2/1 -> STEAM FLOW RATE/1, Mux/40
  W_db/1 -> Mux/41
  W_b/1 -> Mux/42
  Unit Delay4/1 -> To Workspace/1

== system MSDR_and_BOP_v1_1/SECONDARY SIDE/OTSG + BALANCE OF PLANT/REHEATER ==
  note: Rate of change of volumetric density of steam in reheater
  note: Enthalpy of steam in reheater
  note: Steam flow from reheater to LP turbine
  note: Enthalpy of saturated vapor as a function of reheater pressure
  note: Flow from reheater to feedwater heater 2
  note: Heat transfer rate in the reheater
  note: Temperature of shell side steam in reheater
  note: # keeping same density, doubled volume
  note: #doubled volume means double residence time
  note: #doubled volume means double residence time
  STEAM FLOW RATE - SECONDARY VALVE : Inport
  FLOW from MOISTURE SEPARATOR : Inport  Port=2
  STEAM TEMPERATURE : Inport  Port=3
  H_g : Fcn  Expr=u[7]
  H_rh : Integrator  InitialCondition=H_rh
  Mux : Mux  Inputs=12
      settings: DisplayOption=signals
  Q_rh : Integrator  InitialCondition=Q_rh
  RH H_liq : Lookup_n-D  NumberOfTableDimensions=1  BreakpointsForDimension1=P_rh_table1  Table=H_rh_table1  InternalRulePriority=Speed  RndMeth=Simplest  InputSameDT=on
  RH Pressure : Lookup_n-D  BreakpointsForDimension1=H_rh_table2  BreakpointsForDimension2=rho_rh_table  Table=P_rh_table  InternalRulePriority=Speed  RndMeth=Simplest  InputSameDT=on
  RH density : Fcn  Expr=u[5]
  RH enthalpy : Fcn  Expr=u[6]
  T_rh : Fcn  Expr=u[7]*0.75*M_stm/(u[5]*R)
  To Workspace : ToWorkspace  VariableName=RH_mux  SampleTime=0.1
      settings: Save2DSignal=2-D array (concatenate along first dimension)
  Unit Delay1 : UnitDelay  InitialCondition=203.11  SampleTime=-1  HasFrameUpgradeWarning=on
  Unit Delay2 : UnitDelay  InitialCondition=2.8029  SampleTime=-1  HasFrameUpgradeWarning=on
  Unit Delay3 : UnitDelay  InitialCondition=466.87  SampleTime=-1  HasFrameUpgradeWarning=on
  Unit Delay7 : UnitDelay  InitialCondition=2.8582  SampleTime=-1  HasFrameUpgradeWarning=on
  d(H_rh)/dt : Fcn  Expr=(u[11] + u[2]*u[9] - u[8]*u[6])/(u[5]*V_rh) + u[7]*(u[2] - u[8])/(u[5]^2*V_rh)
  d(Q_rh)/dt : Fcn  Expr=((u[1] + u[10])*Cp_hr*(u[3] - u[12]))/(2*tau_rhh) - u[11]/(tau_rhh)
  d(rho_rh)/dt : Fcn  Expr=(u[2] - u[8])/(V_rh)
  d(w'_rh_fwh2)/dt : Fcn  Expr=(u[1] - u[10])/(tau_rh1)
  rho_rh : Integrator  InitialCondition=rho_rh
  w'_rh_fwh2 : Integrator  InitialCondition=51.447
  w_3 : Fcn  Expr=33*(u[7]*u[5])^0.5
  "FLOW to LP TURBINE " : Outport
  FLOW to FWH2 : Outport  Port=2
  STEAM PRESSURE - REHEATER : Outport  Port=3
  STEAM ENTHALPY - REHEATER : Outport  Port=4
  wires:
  STEAM FLOW RATE - SECONDARY VALVE/1 -> Mux/1
  FLOW from MOISTURE SEPARATOR/1 -> Mux/2
  STEAM TEMPERATURE/1 -> Mux/3
  H_rh/1 -> STEAM ENTHALPY - REHEATER/1, Mux/6
  d(H_rh)/dt/1 -> H_rh/1
  rho_rh/1 -> Mux/5
  d(rho_rh)/dt/1 -> rho_rh/1, Mux/4
  Unit Delay7/1 -> Mux/7, STEAM PRESSURE - REHEATER/1
  RH density/1 -> RH Pressure/2
  RH Pressure/1 -> Unit Delay7/1
  RH enthalpy/1 -> RH Pressure/1
  Unit Delay1/1 -> "FLOW to LP TURBINE "/1, Mux/8
  w_3/1 -> Unit Delay1/1
  H_g/1 -> RH H_liq/1
  Unit Delay2/1 -> Mux/9
  d(w'_rh_fwh2)/dt/1 -> w'_rh_fwh2/1
  w'_rh_fwh2/1 -> FLOW to FWH2/1, Mux/10
  d(Q_rh)/dt/1 -> Q_rh/1
  Q_rh/1 -> Mux/11
  T_rh/1 -> Unit Delay3/1
  Mux/1 -> To Workspace/1, T_rh/1, d(Q_rh)/dt/1, d(w'_rh_fwh2)/dt/1, H_g/1, w_3/1, RH enthalpy/1, d(H_rh)/dt/1, d(rho_rh)/dt/1, RH density/1
  RH H_liq/1 -> Unit Delay2/1
  Unit Delay3/1 -> Mux/12

== system MSDR_and_BOP_v1_1/SECONDARY SIDE/OTSG + BALANCE OF PLANT/SECONDARY STEAM VALVE ==
  STEAM FROM OTSG : Inport
  Product : Product
  SSV Coefficient 16% diverted to reheater : Constant  Value=.16
  STEAM TO REHEATER : Outport
  wires:
  STEAM FROM OTSG/1 -> Product/2
  Product/1 -> STEAM TO REHEATER/1
  SSV Coefficient 16% diverted to reheater/1 -> Product/1

== system MSDR_and_BOP_v1_1/SECONDARY SIDE/OTSG + BALANCE OF PLANT/Subsystem ==
  Add : Sum
  Ramp : simulink/Sources/Ramp  slope=0.01/60  start=1000  InitialOutput=1
  Ramp1 : simulink/Sources/Ramp  slope=.1/60  start=3600  InitialOutput=0
  Saturation : Saturate  UpperLimit=1.1  LowerLimit=.5
  Saturation1 : Saturate  UpperLimit=.5  LowerLimit=0
  Out1 : Outport
  wires:
  Saturation/1 -> Add/1
  Saturation1/1 -> Add/2
  Ramp1/1 -> Saturation1/1
  Ramp/1 -> Saturation/1
  Add/1 -> Out1/1
